simulink model "example_HeatPump_conf"  (R2013b)
settings: Solver=ode45  StartTime=0.0  StopTime=1*24*3600  RelTol=1e-4  AbsTol=1e-5
libraries: carnot x6, simulink x1
settings Model: Creator=drhf  LastModifiedBy=drhf
settings OptimizationCC: ExpressionDepthLimit=2147483647
settings DebuggingCC: StateNameClashWarn=warning
settings GRTTargetCC: CombineOutputUpdateFcns=off  GRTInterface=on

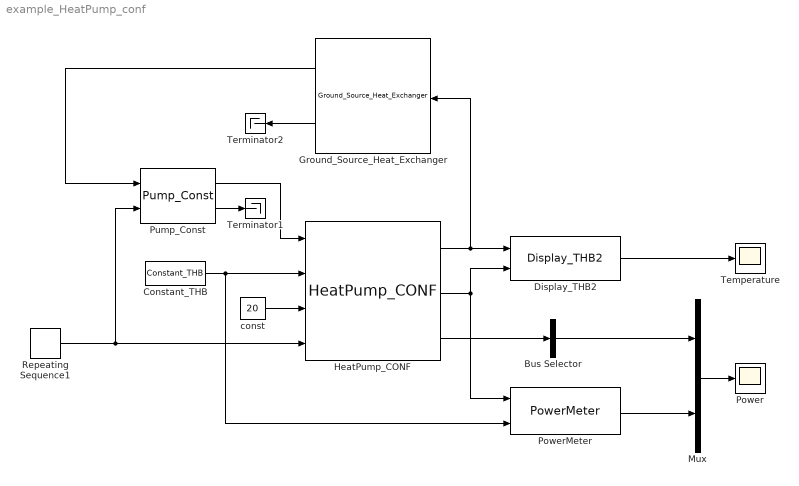
== system example_HeatPump_conf ==
  Bus Selector : BusSelector  OutputSignals=Pelec,Qdot_cold,Qdot_hot  OutputAsBus=on
  Constant_THB : carnot/Source/Simple/Constant_THB  t=40  mdot=2000/3600  p=1e5  mID=No Pressure Drop  fluid=Water  mix=0  mix2=0  mix3=0  dia=0.02  hgt=0
  Display_THB2 : carnot/Outputs/Display_THB2  t=on  m=off  p=off  id=off  mix=off  d=off
  Ground_Source_Heat_Exchanger : carnot/Source/Heat_Pump/Ground_Source_Heat_Exchanger  Jahresmitteltemp_C=12  TGrad=0.025  lambdaErde=2.0  cpErde=800  rhoErde=2500  lambdaFill=1.0  cpFill=1000  rhoFill=2000  Sondelaenge=100  B=10  Sondendurchmesser=0.032  Bohrdurchmesser=0.18  sondenfall=2 probes B/H = 0.1  np=2  DimAxi=10  DimRad=10  Gitterfaktor=2.5
  HeatPump_CONF : carnot/Source/Heat_Pump/HeatPump_CONF  parameterfile=DefaultHeatPump
  Mux : Mux  Inputs=2
  Power : Scope
      settings: TickLabels=on  YMin=-20000  YMax=20000
  PowerMeter : carnot/Control/PowerMeter
  Pump_Const : carnot/Hydraulics/Pump_Const  mdotmax=3000/3600  dia=0.0157  power=30  p0=3e5  fluid_id=Water  mix=0  UA=3  mcp=4000  tamb=20
  Repeating Sequence1 : simulink/Sources/Repeating Sequence  rep_seq_t=[0 0.5 1.5 2]*3600  rep_seq_y=[0 1 1 0]
  Temperature : Scope
      settings: TickLabels=on  YMin=-20  YMax=50
  Terminator1 : Terminator
  Terminator2 : Terminator
  const : Constant  Value=20
  wires:
  Repeating Sequence1/1 -> Pump_Const/2, HeatPump_CONF/4
  Display_THB2/1 -> Temperature/1
  Mux/1 -> Power/1
  PowerMeter/1 -> Mux/2
  Bus Selector/1 -> Mux/1
  HeatPump_CONF/3 -> Bus Selector/1
  HeatPump_CONF/1 -> Ground_Source_Heat_Exchanger/1, Display_THB2/1
  HeatPump_CONF/2 -> Display_THB2/2, PowerMeter/1
  const/1 -> HeatPump_CONF/3
  Constant_THB/1 -> PowerMeter/2, HeatPump_CONF/2
  Pump_Const/1 -> HeatPump_CONF/1
  Pump_Const/2 -> Terminator1/1
  Ground_Source_Heat_Exchanger/2 -> Terminator2/1
  Ground_Source_Heat_Exchanger/1 -> Pump_Const/1
